simulink model "GFLIB_Lut2D_BAM_F16"  (Simulink 8.3)
settings: Solver=ode45  StartTime=0.0  StopTime=10.0  RelTol=1e-3
undefined symbols (not defined in the file): pf16Table, s16MidIdx, u16ShamOffset1, u16ShamOffset2
settings Model: Creator=B17364  LastModifiedBy=B17364
settings OptimizationCC: ExpressionDepthLimit=2147483647
settings DebuggingCC: FcnCallInpInsideContextMsg=UseLocalSettings  StrictBusMsg=Warning

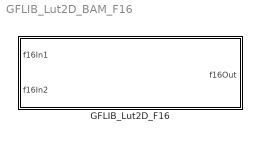
== system GFLIB_Lut2D_BAM_F16 ==
  GFLIB_Lut2D_F16 : Subsystem  mask(GFLIB_Lut2D_F16){u16ShamOffset1=u16ShamOffset1, u16ShamOffset2=u16ShamOffset2, pf16Table=pf16Table, s16MidIdx=s16MidIdx}
      mask help: Bit accurate model of Lut2D function.
      mask init:
      | pos = get_param(gcb, 'Position');width = pos(3) - pos(1); height = pos(4) - pos(2);tX=width/2;tY=height*0.9;
      mask Display: color('black');port_label('input',1,'f16In1');port_label('input',2,'f16In2');port_label('output',1,'f16Out');color('black');disp('GFLIB_Lut2D_F16');color('blue');text(tX,tY, 'BAM', 'horizontalAlignment', 'center');

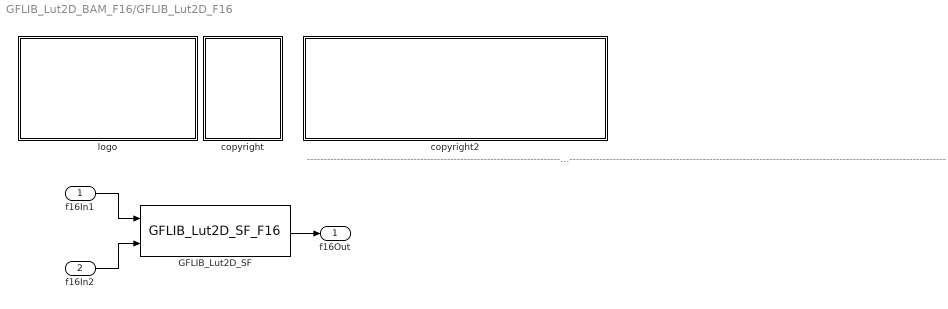
== system GFLIB_Lut2D_BAM_F16/GFLIB_Lut2D_F16 ==
  note: ---------------------------------------------------------------------------------------------------------------------------------------------------------------------------------------------------
  f16In1 : Inport
  f16In2 : Inport  Port=2
  GFLIB_Lut2D_SF : S-Function  FunctionName=GFLIB_Lut2D_SF_F16  Parameters=u16ShamOffset1,u16ShamOffset2,pf16Table,s16MidIdx  EnableBusSupport=off
  copyright : Subsystem
      mask Display:
      | text(10,90,'FILE:');text(10,75,'DESRIPTION:')
      | text(10,60,'COPYRIGHT:')
      | text(10,45,'VERSION:')
      | text(10,30,'DATE:')
  copyright2 : Subsystem
      mask Display:
      | text(10,90,'GFLIB_Lut2D_BAM_F16.mdl');text(10,75,'Two dimensional Look-up table function');text(10,60,'Freescale')
      | text(10,45,'0.1');text(10,30,'17-Jun-2013');
  logo : Subsystem
      mask Display: image(imread('logo.jpg'))
  f16Out : Outport
  wires:
  f16In1/1 -> GFLIB_Lut2D_SF/1
  f16In2/1 -> GFLIB_Lut2D_SF/2
  GFLIB_Lut2D_SF/1 -> f16Out/1

== system GFLIB_Lut2D_BAM_F16/GFLIB_Lut2D_F16/copyright ==

== system GFLIB_Lut2D_BAM_F16/GFLIB_Lut2D_F16/copyright2 ==

== system GFLIB_Lut2D_BAM_F16/GFLIB_Lut2D_F16/logo ==
